simulink model "twotone_amp"  (Simulink 6.0)
settings: Solver=ode45  StartTime=0.0  StopTime=10.0  RelTol=1e-3
undefined symbols (not defined in the file or in its folder): dTypeID, Fs, read, rfdata
libraries: dspsnks4 x2, rfports1 x2, dspmtrx3 x1, simulink x1, rfamplifiers1 x1
settings Model: Creator=ashivapr  LastModifiedBy=rzeng  ExtModeAutoUpdateStatusClock=off  ProdHWDeviceType=Specified
settings DataIOCC: SaveOutput=off  SaveTime=off  SignalLoggingName=logsOut
settings DebuggingCC: CheckExecutionContextPreStartOutputMsg=on  CheckExecutionContextRuntimeOutputMsg=on  SolverPrmCheckMsg=none
settings HardwareCC: ProdHWDeviceType=Specified
settings ModelReferenceCC: UpdateModelReferenceTargets=IfOutOfDate
settings SFSimCC: SFSimApplyToAllLibs=on  SFSimBuildMode=Incremental

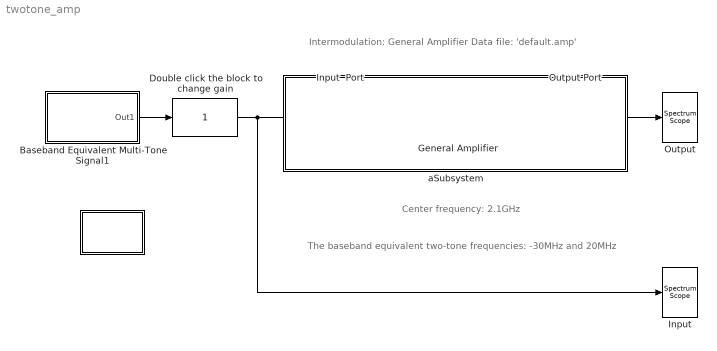
== system twotone_amp ==
  note: Intermodulation: General Amplifier
      | Data file: 'default.amp'
  note: Center frequency: 2.1GHz
  note: The baseband equivalent
      |  two-tone frequencies:
      | -30MHz and 20MHz
  " " : Subsystem  PropExecContextAcrossSSBoundary=on
      mask Type: Interpolation filter info block
      mask Display: disp('Info')
  Baseband Equivalent Multi-Tone Signal1 : Subsystem  PropExecContextAcrossSSBoundary=on  mask(Baseband Equivalent Multi-Tone Sine Wave){Fc=2.1e9, Frequency=[2.07e9 2.12e9], Amplitude=[0.1 0.05], Phase=[0 pi/4], SampleTime=3e-9, SamplesPerFrame=256}
      mask prompts: Fc "Center frequency (Hz)"; Frequency "Tone frequency (Hz):"; Amplitude "Tone amplitude:"; Phase "Tone phase offset (rad):"; SampleTime "Sample time:"; SamplesPerFrame "Samples per frame:"
      mask help:
      | Generate a baseband equivalent multi-tone complex sinusoid signal. The frequency of the output multi-tone signal is the difference between the Tone frequency and the Center frequency.
      |
      | The values specified here for the Center frequency and Sample time parameters should be equal to the values specified in the 'Input Port' block.
      mask init:
      | if ~isscalar(Fc)
      | 	error('Center frequency must be a scalar');
      | end
      | if ~isnumeric(Frequency)
      | 	error('Tone frequency must be a real vector');
      | end
      | if any(Frequency>=2*Fc)
      | 	error('Tone frequency is too large compared to the Center frequency');
      | end
      | 
      | Frequency = Frequency-Fc;
      mask Display:
      | plot(-0.5,-3,1.5,1,[0:0.005:1], [0.25*sin(2*pi*5*[0:0.005:1])+0.5*sin(2*pi*10*[0:0.005:1]) ]);
      | disp('\nMulti-Tone');
  Double click the block to change gain : simulink/Math Operations/Slider Gain  low=1  gain=1  high=10
  General Amplifier : rfamplifiers1/General Amplifier  PhysicalDomain=rfsystemsdomain  SubClassName=general-amplifier  LeftPortType=p1  RightPortType=p1  LConnTagsString=__newl0  RConnTagsString=__newr0  RFDATA=read(rfdata.data, 'default.amp')  InterpMethod=Cubic  IP3Type=OIP3  IIP3=inf  OIP3=30  NF=0  DisplayData=off  PlotFreq=Derived from Input Port parameters  PlotFreqNoSim=Extracted from RFDATA object  Freq=[1.0e9:1.0e8:2.9e9]  AllPlotType=X-Y plane  NetworkData=S21  PowerData=S11  SmithData=S11  PolarData=S11  ComplexFormat=Magnitude (decibels)  DBFormat=Magnitude (decibels)  PowerFormat=dBm  PhaseFormat=Angle (degrees)  NoneFormat=None
  Input : dspsnks4/Spectrum Scope  ScopeProperties=off  Domain=Frequency  HorizSpan=1  UseBuffer=off  BufferSize=128  Overlap=64  inpFftLenInherit=off  FFTlength=1024  numAvg=20  DisplayProperties=on  AxisGrid=on  Memory=off  FrameNumber=off  AxisLegend=off  AxisZoom=off  OpenScopeAtSimStart=on  OpenScopeImmediately=off  FigPos=[40 296 332 250]  AxisProperties=off  XUnits=Hertz  XRange=[-Fs/2...Fs/2]  InheritXIncr=on  XIncr=1.0  XLabel=Samples  YUnits=dB  YLabel=Magnitude, dB  LineProperties=off
      settings: YMin=-157.530034383769  YMax=3.98302119684644
  Input  Port : rfports1/Input Port  Description=source block  MaxLength=128  Fc=2.1e9  Ts=3e-9  Zs=50  NoiseFlag=off  seed=67987  GoToTag=BBDEHJKPWQQMHEIKGDHPMBF
  Output : dspsnks4/Spectrum Scope  ScopeProperties=off  Domain=Frequency  HorizSpan=1  UseBuffer=off  BufferSize=128  Overlap=64  inpFftLenInherit=off  FFTlength=1024  numAvg=20  DisplayProperties=on  AxisGrid=on  Memory=off  FrameNumber=off  AxisLegend=off  AxisZoom=off  OpenScopeAtSimStart=on  OpenScopeImmediately=off  FigPos=[379 296 350 250]  AxisProperties=off  XUnits=Hertz  XRange=[-Fs/2...Fs/2]  InheritXIncr=on  XIncr=1.0  XLabel=Samples  YUnits=dB  YLabel=Magnitude, dB  LineProperties=off
      settings: YMin=-142.794240384809  YMax=19.9039831433459
  Output Port : rfports1/Output Port  Zl=50  num_Models=3  GoToTag=BBDEHJKPWQQMHEIKGDHPMBF  DisplayData=off  PlotFreq=Derived from Input Port parameters  Freq=1e9:1e8:3e9  AllPlotType=Composite data  NoBudgetPlot=Composite data  NetworkData=S11  SmithData=S11  PolarData=S11  ComplexFormat=Magnitude (decibels)  DBFormat=Magnitude (decibels)  DBMFormat=dBm  NoneFormat=None
  aSubsystem : Subsystem  PropExecContextAcrossSSBoundary=on
      mask Display: disp('')
  wires:
  Baseband Equivalent Multi-Tone Signal1/1(Out1) -> Double click the block to change gain/1
  Output Port/1 -> Output/1
  Double click the block to change gain/1 -> Input  Port/1, Input/1
  connections:
  Input  Port/RConn1 -- General Amplifier/LConn1
  General Amplifier/RConn1 -- Output Port/LConn1

== system twotone_amp/  ==
  note: Intermodulation: General Amplifier
      |
      | The Amplifiers library has blocks to represent
      | amplifiers in terms of S, Y, and Z parameters.
      | The library also has the 'General Amplifier' block
      | that can be used for AMP data file.
      |
      | The data file: 'default.amp' has
      | the S-parameters of an amplifier and its
      | Pin-Pout data at 2.1GHz.
      |
      | To view the intermodulation performance at the output,
      | double click the 'Slider Gain' block and change the gain
      | while the model is running.
      |
      | To compare with the intermodulation of mathematical
      | amplifier, simulate the demo:
      | Comparison of Amplifiers: Linear vs Nonlinear.

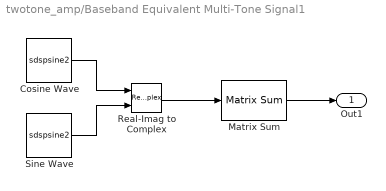
== system twotone_amp/Baseband Equivalent Multi-Tone Signal1 ==
  Cosine Wave : S-Function  AncestorBlock=dspsrcs4/Sine Wave  FunctionName=sdspsine2  Parameters=Amplitude,Frequency,Phase,SampleMode,OutComplex,CompMethod,SampleTime,SamplesPerFrame,ResetState,TableSize,isCustomFloat,isSigned,dTypeID,wordLength,fracBits  mask(Sine Wave){Amplitude=Amplitude, Frequency=Frequency, Phase=Phase+(pi/2), SampleMode=Discrete, OutComplex=Real, CompMethod=Trigonometric fcn, TableSize=Speed, SampleTime=SampleTime, SamplesPerFrame=SamplesPerFrame, additionalParams=off, allowOverrides=on, dataType=double, wordLen=16, udDataType=sfix(16), fracBitsMode=Best precision, numFracBits=15, ResetState=Restart at time zero}
      mask prompts: Frequency "Frequency (Hz):"; Phase "Phase offset (rad):"; SampleMode "Sample mode:"; OutComplex "Output complexity:"; CompMethod "Computation method:"; TableSize "Optimize table for:"; SampleTime "Sample time:"; SamplesPerFrame "Samples per frame:"; additionalParams "------- Show additional parameters --------"; allowOverrides "Allow overrides from DSP Fixed-Point Attributes blocks"; dataType "Output data type:"; wordLen "Word length:"; udDataType "User-defined data type (e.g. sfix(16), float('single')):"; fracBitsMode "Set fraction length in output to:"; numFracBits "Fraction length:"; ResetState "State when re-enabled:"
      mask help: Output samples of a sinusoid. To generate more than one sinusoid simultaneously, enter a vector of values for the amplitude, frequency, and phase parameters.
      mask init:
      | [x,y] = dspblksine('icon');
      | [dtInfo,dTypeID]=dspblksine('init');
      | isSigned=dtInfo.DataTypeIsSigned;
      | isCustomFloat=dtInfo.DataTypeIsCustomFloat;
      | wordLength=dtInfo.DataTypeWordLength;
      | fracBits=dtInfo.DataTypeFracOrMantBits;
      | dType=dataType;
      mask Help: web(dspbhelp);
      mask StyleString: edit,edit,edit,popup(Discrete|Continuous),popup(Real|Complex),popup(Trigonometric fcn|Table lookup|Differential),popup(Speed|Memory),edit,edit,checkbox,checkbox,popup(double|single|Fixed-point|User-defined|Inherit via back propagation),edit,edit,popup(Best precision|User-defined),edit,popup(Restart at time zero|Catch up to simulation time)
      mask CallbackString: |||dspblksine;||dspblksine;||||dspblksine|dspblksine|dspblksine||dspblksine|dspblksine||
      mask Display:
      | plot(x,y)
      | text(3.25,.75,'DSP');
  Matrix Sum : dspmtrx3/Matrix Sum  DialogController=dspDDGCreate  DialogControllerArgs=DataTag0  Dim=Rows  roundingMode=Floor  overflowMode=off
  Real-Imag to Complex : RealImagToComplex
  Sine Wave : S-Function  AncestorBlock=dspsrcs4/Sine Wave  FunctionName=sdspsine2  Parameters=Amplitude,Frequency,Phase,SampleMode,OutComplex,CompMethod,SampleTime,SamplesPerFrame,ResetState,TableSize,isCustomFloat,isSigned,dTypeID,wordLength,fracBits  mask(Sine Wave){Amplitude=Amplitude, Frequency=Frequency, Phase=Phase, SampleMode=Discrete, OutComplex=Real, CompMethod=Trigonometric fcn, TableSize=Speed, SampleTime=SampleTime, SamplesPerFrame=SamplesPerFrame, additionalParams=off, allowOverrides=on, dataType=double, wordLen=16, udDataType=sfix(16), fracBitsMode=Best precision, numFracBits=15, ResetState=Restart at time zero}
      mask prompts: Frequency "Frequency (Hz):"; Phase "Phase offset (rad):"; SampleMode "Sample mode:"; OutComplex "Output complexity:"; CompMethod "Computation method:"; TableSize "Optimize table for:"; SampleTime "Sample time:"; SamplesPerFrame "Samples per frame:"; additionalParams "------- Show additional parameters --------"; allowOverrides "Allow overrides from DSP Fixed-Point Attributes blocks"; dataType "Output data type:"; wordLen "Word length:"; udDataType "User-defined data type (e.g. sfix(16), float('single')):"; fracBitsMode "Set fraction length in output to:"; numFracBits "Fraction length:"; ResetState "State when re-enabled:"
      mask help: Output samples of a sinusoid. To generate more than one sinusoid simultaneously, enter a vector of values for the amplitude, frequency, and phase parameters.
      mask init: same as twotone_amp/Baseband Equivalent Multi-Tone Signal1/Cosine Wave
      mask Help: web(dspbhelp);
      mask StyleString: edit,edit,edit,popup(Discrete|Continuous),popup(Real|Complex),popup(Trigonometric fcn|Table lookup|Differential),popup(Speed|Memory),edit,edit,checkbox,checkbox,popup(double|single|Fixed-point|User-defined|Inherit via back propagation),edit,edit,popup(Best precision|User-defined),edit,popup(Restart at time zero|Catch up to simulation time)
      mask CallbackString: |||dspblksine;||dspblksine;||||dspblksine|dspblksine|dspblksine||dspblksine|dspblksine||
      mask Display:
      | plot(x,y)
      | text(3.25,.75,'DSP');
  Out1 : Outport
  wires:
  Matrix Sum/1 -> Out1/1
  Cosine Wave/1 -> Real-Imag to Complex/1
  Sine Wave/1 -> Real-Imag to Complex/2
  Real-Imag to Complex/1 -> Matrix Sum/1

== system twotone_amp/aSubsystem ==
